simulink model "Studio6_1_2018b"  (R2020a)
settings: Solver=ode45  StartTime=0.  StopTime=80  FixedStep=0.2  MaxStep=0.05  RelTol=1e-8  AbsTol=1e-8  EnableMultiTasking=on
settings Model: ExtModeTrigMode=oneshot  ExtModeArmWhenConnect=off  Creator=LEVIENKL  LastModifiedBy=Vy Possible
settings SolverCC: AutoScaleAbsTol=off
settings DataIOCC: SaveFormat=Array  SignalLoggingSaveFormat=ModelDataLogs  SaveOutput=off  SaveTime=off  ReturnWorkspaceOutputs=off  SignalLoggingName=sigsOut
settings OptimizationCC: BlockReduction=off  BooleanDataType=off  ExpressionDepthLimit=2147483647  InitFltsAndDblsToZero=on  LifeSpan=inf
settings DebuggingCC: SaveWithParameterizedLinksMsg=none  UnderspecifiedInitializationDetection=Classic  MergeDetectMultiDrivingBlocksExec=none  SignalResolutionControl=TryResolveAllWithWarning  MultiTaskDSMMsg=warning  MultiTaskCondExecSysMsg=none  FcnCallInpInsideContextMsg=warning  AllowSymbolicDim=off  StateNameClashWarn=warning  SFUnexpectedBacktrackingDiag=warning  SFNoUnconditionalDefaultTransitionDiag=warning  SFExecutionAtInitializationDiag=none  ArithmeticOperatorsInVariantConditions=warning
settings HardwareCC: ProdBitPerPointer=32  ProdBitPerSizeT=32  ProdBitPerPtrDiffT=32  ProdLargestAtomicFloat=None  ProdIntDivRoundTo=Undefined  ProdEndianess=Unspecified  ProdWordSize=32  ProdHWDeviceType=32-bit Generic  TargetUnknown=on
settings ModelReferenceCC: PropagateSignalLabelsOutOfModel=off
settings SFSimCC: SimUseLocalCustomCode=off  CustomCodeUndefinedFunction=UseInterfaceOnly
settings RTWCC: RTWUseLocalCustomCode=off
settings CodeAppCC: StateflowObjectComments=on
settings GRTTargetCC: TargetFcnLib=ansi_tfl_tmw.mat  TargetLangStandard=C89/C90 (ANSI)  CombineOutputUpdateFcns=off  GRTInterface=on
settings ConfigComp: CovMetricSettings=dw  CovHtmlReporting=on  CovSaveCumulativeToWorkspaceVar=on  CovSaveSingleToWorkspaceVar=on  CovExternalEMLEnable=off  CovSFcnEnable=off

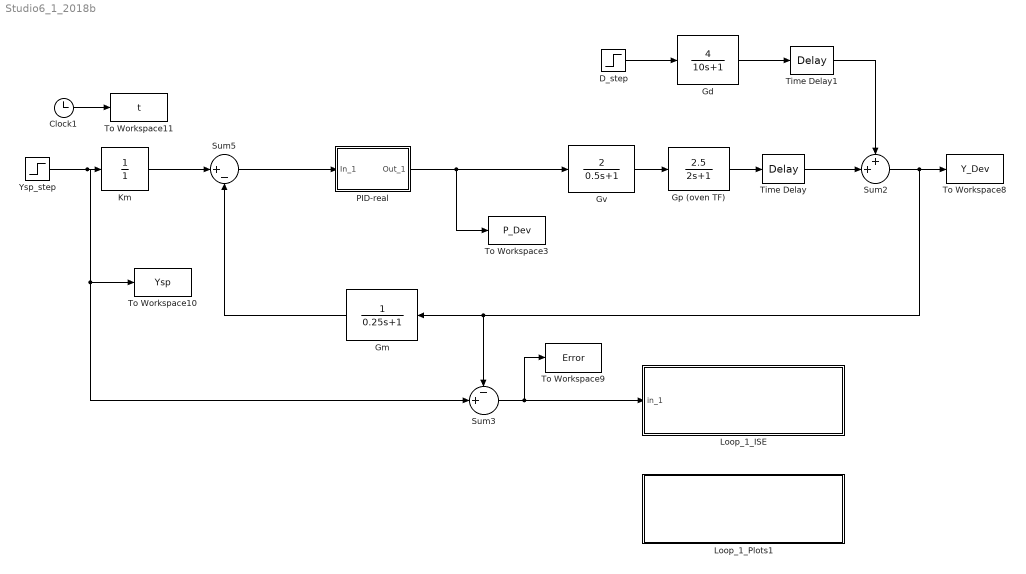
== system Studio6_1_2018b ==
  Clock1 : Clock
  D_step : Step  Time=5  After=0  SampleTime=0
      settings: AttributesFormatString=%<Before> to %<After>\nat %<Time>
  Gd : TransferFcn  Numerator=[4]  Denominator=[10 1]
  Gm : TransferFcn  Denominator=[0.25 1]
  Gp (oven TF) : TransferFcn  Numerator=[2.5]  Denominator=[2 1]
  Gv : TransferFcn  Numerator=[2]  Denominator=[0.5 1]
  "Km " : TransferFcn  Denominator=[0 1]
  Loop_1_ISE : Subsystem  mask(Integral Squarred Evaluation - Loop 1){}
      settings: OpenFcn=ISE1
      mask Help: This block calculates and plots loop #1 ISE.
      mask Display: disp('After Loop 1 Simulation:\n Double Click for ISE evaluation\n (uses ISE1.p)')
  Loop_1_Plots1 : Subsystem  mask(Y,U,E Plots - Loop 1){}
      settings: OpenFcn=YPEplots
      mask Help: This block loop #1 Y,U,Error in 3x1 Figure Window.
      mask Display: disp('After Loop 1 Simulation:\n Double Click for Y, P, Error Plots\n (uses YPEplots.p)')
  PID-real : Subsystem  mask(PID(with alpha) Controller for ChE 461){Kc=0.2, tauIi=1/2, tauD=0.5, alpha=0.05}
      mask prompts: Kc "Controller gain:"; tauIi "Inv of Integral time constant (careful - this is I action ! ) :"; tauD "Derivative time constant:"; alpha "Alpha value (small)::"
      mask help:
      | Enter expressions for controller gain,
      | inverse of integral time constant
      | and derivative time constant and alpha.
      settings: AttributesFormatString=Kc = %<Kc>\n1/TauI = %<tauIi>\nTauD = %<tauD>
      mask Help: This block implements a PID controller where parameters are entered for the Controller Gain, inverse of Integral time constant and Derivative time constant.  Alpha here is equal to 0.01.   Unmask this block to see how it works. The derivative term is implemented using a true derivative block.
      mask Display: disp('PIDalpha')
  Sum2 : Sum  Inputs=++|  InputSameDT=on  SaturateOnIntegerOverflow=on  OutDataTypeStr=Inherit: Same as first input
  Sum3 : Sum  Inputs=-+|  InputSameDT=on  SaturateOnIntegerOverflow=on  OutDataTypeStr=Inherit: Same as first input
  Sum5 : Sum  Inputs=|+-  InputSameDT=on  SaturateOnIntegerOverflow=on  OutDataTypeStr=Inherit: Same as first input
  Time Delay : TransportDelay  DelayTime=0.2
      settings: AttributesFormatString=Delay=%<DelayTime>
  Time Delay1 : TransportDelay  DelayTime=0.2
      settings: AttributesFormatString=Delay=%<DelayTime>
  To Workspace10 : ToWorkspace  VariableName=Ysp  SampleTime=-1
  To Workspace11 : ToWorkspace  VariableName=t  SampleTime=-1
  To Workspace3 : ToWorkspace  VariableName=P_Dev  SampleTime=-1
  To Workspace8 : ToWorkspace  VariableName=Y_Dev  SampleTime=-1
  To Workspace9 : ToWorkspace  VariableName=Error  SampleTime=-1
  Ysp_step : Step  Time=5  After=10  SampleTime=0
      settings: AttributesFormatString=%<Before> to %<After>\nat %<Time>
  wires:
  Ysp_step/1 -> "Km "/1, Sum3/2, To Workspace10/1
  PID-real/1(Out_1) -> Gv/1, To Workspace3/1
  "Km "/1 -> Sum5/1
  Clock1/1 -> To Workspace11/1
  Sum3/1 -> To Workspace9/1, Loop_1_ISE/1(in_1)
  Gm/1 -> Sum5/2
  Gv/1 -> Gp (oven TF)/1
  D_step/1 -> Gd/1
  Gd/1 -> Time Delay1/1
  Time Delay1/1 -> Sum2/1
  Gp (oven TF)/1 -> Time Delay/1
  Time Delay/1 -> Sum2/2
  Sum2/1 -> Gm/1, Sum3/1, To Workspace8/1
  Sum5/1 -> PID-real/1(In_1)

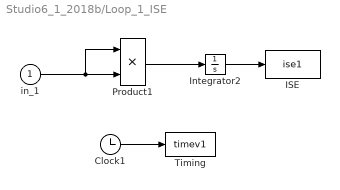
== system Studio6_1_2018b/Loop_1_ISE ==
  in_1 : Inport
  Clock1 : Clock
  ISE : ToWorkspace  VariableName=ise1
      settings: MaxDataPoints=20000
  Integrator2 : Integrator
  Product1 : Product  InputSameDT=on  RndMeth=Zero  SaturateOnIntegerOverflow=on  OutDataTypeStr=Inherit: Same as first input
  Timing : ToWorkspace  VariableName=timev1
      settings: MaxDataPoints=20000
  wires:
  in_1/1 -> Product1/2, Product1/1
  Integrator2/1 -> ISE/1
  Clock1/1 -> Timing/1
  Product1/1 -> Integrator2/1

== system Studio6_1_2018b/Loop_1_Plots1 ==

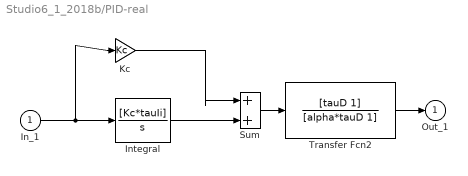
== system Studio6_1_2018b/PID-real ==
  In_1 : Inport
  Integral : TransferFcn  Numerator=[Kc*tauIi]  Denominator=[1 0]
  Kc : Gain  Gain=Kc  SaturateOnIntegerOverflow=on  OutDataTypeStr=Inherit: Same as input  ParamDataTypeStr=Inherit: Same as input
  Sum : Sum  InputSameDT=on  SaturateOnIntegerOverflow=on  OutDataTypeStr=Inherit: Same as first input
  Transfer Fcn2 : TransferFcn  Numerator=[tauD 1]  Denominator=[alpha*tauD 1]
  Out_1 : Outport  VectorParamsAs1DForOutWhenUnconnected=off
  wires:
  Transfer Fcn2/1 -> Out_1/1
  Sum/1 -> Transfer Fcn2/1
  In_1/1 -> Integral/1, Kc/1
  Integral/1 -> Sum/2
  Kc/1 -> Sum/1
